simulink model "pole"  (R2020b)
settings: Solver=VariableStepAuto  StartTime=0.0  StopTime=10.0  RelTol=1e-3
libraries: cstblocks x6
settings Model: Creator=Mah  LastModifiedBy=Mah

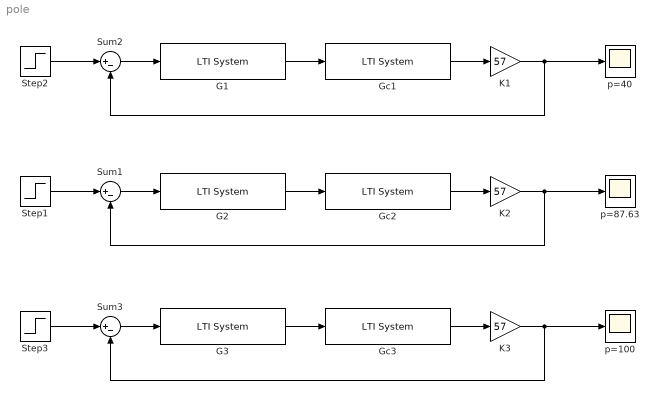
== system pole ==
  G1 : cstblocks/LTI System  sys=tf(64.11 , [1 36.42 0])  IC=[]
  G2 : cstblocks/LTI System  sys=tf(64.11 , [1 36.42 0])  IC=[]
  G3 : cstblocks/LTI System  sys=tf(64.11 , [1 36.42 0])  IC=[]
  Gc1 : cstblocks/LTI System  sys=tf([1 40] , [1 40])  IC=[]
  Gc2 : cstblocks/LTI System  sys=tf([1 40] , [1 87.6383])  IC=[]
  Gc3 : cstblocks/LTI System  sys=tf([1 40] , [1 100])  IC=[]
  K1 : Gain  Gain=57
  K2 : Gain  Gain=57
  K3 : Gain  Gain=57
  Step1 : Step  Time=0  SampleTime=0
  Step2 : Step  Time=0  SampleTime=0
  Step3 : Step  Time=0  SampleTime=0
  Sum1 : Sum  Inputs=|+-
  Sum2 : Sum  Inputs=|+-
  Sum3 : Sum  Inputs=|+-
  p=100 : Scope
  p=40 : Scope
  p=87.63 : Scope
  wires:
  Sum1/1 -> G2/1
  Gc2/1 -> K2/1
  G2/1 -> Gc2/1
  K2/1 -> p=87.63/1, Sum1/2
  Step1/1 -> Sum1/1
  Sum2/1 -> G1/1
  Gc1/1 -> K1/1
  G1/1 -> Gc1/1
  K1/1 -> p=40/1, Sum2/2
  Step2/1 -> Sum2/1
  Sum3/1 -> G3/1
  Gc3/1 -> K3/1
  G3/1 -> Gc3/1
  K3/1 -> p=100/1, Sum3/2
  Step3/1 -> Sum3/1
